simulink library "A_N_to_L"  (R2020b)
settings: Solver=VariableStepAuto  StartTime=0.0  StopTime=10.0  RelTol=1e-3
libraries: vrlib x5
settings Model: Creator=whitehole  LastModifiedBy=whitehole

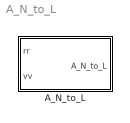
== system A_N_to_L ==
  A_N_to_L : Subsystem

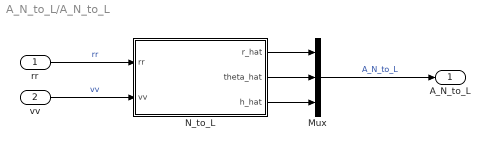
== system A_N_to_L/A_N_to_L ==
  rr : Inport
  vv : Inport  Port=2
  Mux : Mux  Inputs=3
  N_to_L : Subsystem
  A_N_to_L : Outport
  wires:
  rr/1 -> N_to_L/1(rr)  "rr"
  vv/1 -> N_to_L/2(vv)  "vv"
  N_to_L/1(r_hat) -> Mux/1
  N_to_L/2(theta_hat) -> Mux/2
  N_to_L/3(h_hat) -> Mux/3
  Mux/1 -> A_N_to_L/1  "A_N_to_L"

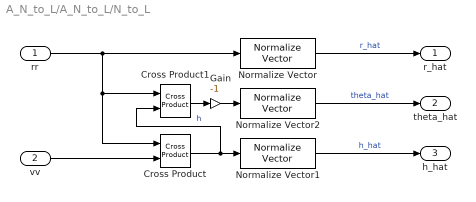
== system A_N_to_L/A_N_to_L/N_to_L ==
  rr : Inport
  vv : Inport  Port=2
  Cross Product : vrlib/Utilities/Cross Product
  Cross Product1 : vrlib/Utilities/Cross Product
  Gain : Gain  Gain=-1
  Normalize Vector : vrlib/Utilities/Normalize Vector  maxzero=0
  Normalize Vector1 : vrlib/Utilities/Normalize Vector  maxzero=0
  Normalize Vector2 : vrlib/Utilities/Normalize Vector  maxzero=0
  r_hat : Outport
  theta_hat : Outport  Port=2
  h_hat : Outport  Port=3
  wires:
  Cross Product1/1 -> Gain/1
  Gain/1 -> Normalize Vector2/1
  Normalize Vector1/1 -> h_hat/1  "h_hat"
  Cross Product/1 -> Cross Product1/2, Normalize Vector1/1  "h"
  vv/1 -> Cross Product/2
  Normalize Vector2/1 -> theta_hat/1  "theta_hat"
  rr/1 -> Cross Product1/1, Cross Product/1, Normalize Vector/1
  Normalize Vector/1 -> r_hat/1  "r_hat"
